simulink model "SIMULACION_LTI_Aumentado"  (R2023b)
settings: Solver=VariableStepAuto  StartTime=0.0  StopTime=2  RelTol=1e-3
values from neighbouring files (symbols this model uses):
  lambda_m = 0.016    [parametros_proyecto2.m]
  Ld = 6.6e-3    (= 0.0066)    [parametros_proyecto2.m]
  Lls = 0.8e-3    (= 0.0008)    [parametros_proyecto2.m]
  Lq = 5.8e-3    (= 0.0058)    [parametros_proyecto2.m]
  r = 120    [parametros_proyecto2.m]
  Rs_ref = 1.02    [parametros_proyecto2.m]
  Rts_amb = 146.7    [parametros_proyecto2.m]
undefined symbols (not defined in the file or in its folder): b_eq, cts, J_eq, P_p, R_s
settings Model: Creator=ignab  LastModifiedBy=ignab

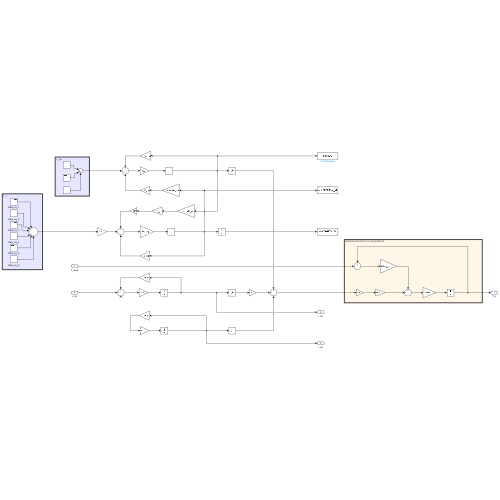
[thumbnail: Simulink's stored preview of the top-level diagram]
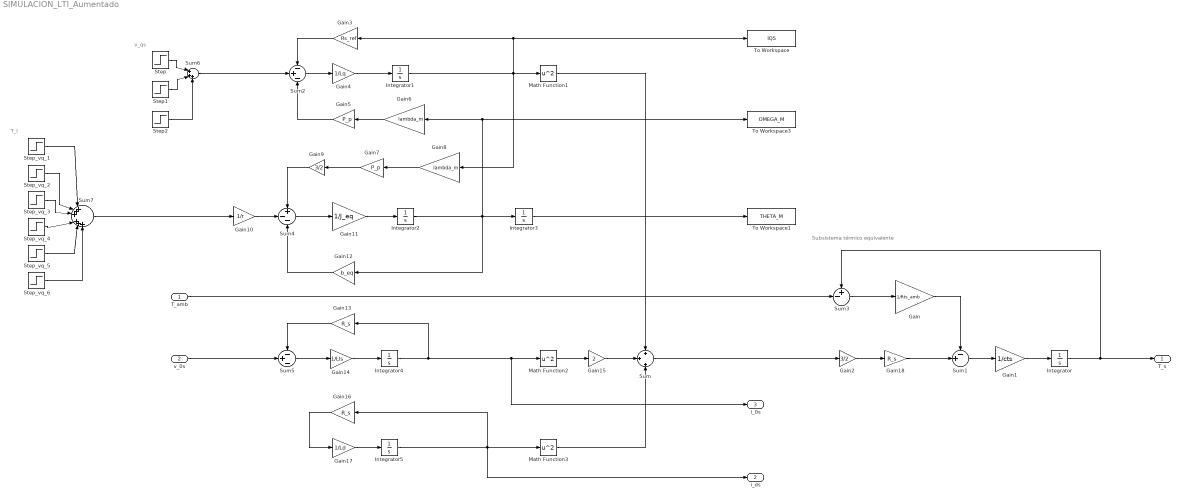
== system SIMULACION_LTI_Aumentado ==
  note: T_l
  note: v_qs
  note: Subsistema térmico equivalente
  T_amb : Inport
  v_0s : Inport  Port=2
  Gain : Gain  Gain=1/Rts_amb
  Gain1 : Gain  Gain=1/cts
  Gain10 : Gain  Gain=1/r
  Gain11 : Gain  Gain=1/J_eq
  Gain12 : Gain  Gain=b_eq
  Gain13 : Gain  Gain=R_s
  Gain14 : Gain  Gain=1/Lls
  Gain15 : Gain  Gain=2
  Gain16 : Gain  Gain=R_s
  Gain17 : Gain  Gain=1/Ld
  Gain18 : Gain  Gain=R_s
  Gain2 : Gain  Gain=3/2
  Gain3 : Gain  Gain=Rs_ref
  Gain4 : Gain  Gain=1/Lq
  Gain5 : Gain  Gain=P_p
  Gain6 : Gain  Gain=lambda_m
  Gain7 : Gain  Gain=P_p
  Gain8 : Gain  Gain=lambda_m
  Gain9 : Gain  Gain=3/2
  Integrator{,1..5} (6 alike) : Integrator
  Math Function1 : Math  Operator=square
  Math Function2 : Math  Operator=square
  Math Function3 : Math  Operator=square
  Step : Step  Time=0.1  After=19.596  SampleTime=0
  Step1 : Step  Time=0.7  After=-39.192  SampleTime=0
  Step2 : Step  Time=1.1  After=19.596  SampleTime=0
  Step_vq_1 : Step  Time=0.3  After=6.28  SampleTime=0
  Step_vq_2 : Step  Time=0.5  After=-12.59  SampleTime=0
  Step_vq_3 : Step  Time=0.9  After=6.28  SampleTime=0
  Step_vq_4 : Step  Time=1.3  After=6.28  SampleTime=0
  Step_vq_5 : Step  Time=1.5  After=-12.59  SampleTime=0
  Step_vq_6 : Step  Time=1.9  After=6.28  SampleTime=0
  Sum : Sum  Inputs=+|+|+
  Sum1 : Sum  Inputs=-+|
  Sum2 : Sum  Inputs=-+-
  Sum3 : Sum  Inputs=+-|
  Sum4 : Sum  Inputs=+--
  Sum5 : Sum  Inputs=-+-
  Sum6 : Sum  Inputs=|+++
  Sum7 : Sum  Inputs=|+++|+++
  To Workspace : ToWorkspace  VariableName=IQS  SaveFormat=Timeseries  SampleTime=-1
      settings: Decimation=2
  To Workspace1 : ToWorkspace  VariableName=THETA_M  SaveFormat=Timeseries  SampleTime=-1
  To Workspace3 : ToWorkspace  VariableName=OMEGA_M  SaveFormat=Timeseries  SampleTime=-1
  T_s : Outport
  i_ds : Outport  Port=2
  i_0s : Outport  Port=3
  wires:
  T_amb/1 -> Sum3/2
  Sum3/1 -> Gain/1
  Gain/1 -> Sum1/1
  Sum1/1 -> Gain1/1
  Gain1/1 -> Integrator/1
  Integrator/1 -> T_s/1, Sum3/1
  Sum6/1 -> Sum2/2
  Gain5/1 -> Sum2/3
  Gain3/1 -> Sum2/1
  Sum2/1 -> Gain4/1
  Gain4/1 -> Integrator1/1
  Gain6/1 -> Gain5/1
  Integrator1/1 -> To Workspace/1, Gain3/1, Math Function1/1, Gain8/1
  Gain8/1 -> Gain7/1
  Gain7/1 -> Gain9/1
  Gain9/1 -> Sum4/1
  Gain12/1 -> Sum4/3
  Sum4/1 -> Gain11/1
  Gain11/1 -> Integrator2/1
  Integrator2/1 -> Integrator3/1, Gain12/1, To Workspace3/1, Gain6/1
  Gain10/1 -> Sum4/2
  Sum7/1 -> Gain10/1
  Integrator4/1 -> i_0s/1, Math Function2/1, Gain13/1
  v_0s/1 -> Sum5/2
  Sum5/1 -> Gain14/1
  Gain14/1 -> Integrator4/1
  Gain13/1 -> Sum5/1
  Gain17/1 -> Integrator5/1
  Gain16/1 -> Gain17/1
  Integrator5/1 -> Gain16/1, Math Function3/1, i_ds/1
  Math Function2/1 -> Gain15/1
  Gain15/1 -> Sum/2
  Math Function1/1 -> Sum/1
  Math Function3/1 -> Sum/3
  Sum/1 -> Gain2/1
  Gain2/1 -> Gain18/1
  Gain18/1 -> Sum1/2
  Integrator3/1 -> To Workspace1/1
  Step2/1 -> Sum6/3
  Step/1 -> Sum6/1
  Step1/1 -> Sum6/2
  Step_vq_1/1 -> Sum7/1
  Step_vq_2/1 -> Sum7/2
  Step_vq_3/1 -> Sum7/3
  Step_vq_4/1 -> Sum7/4
  Step_vq_5/1 -> Sum7/5
  Step_vq_6/1 -> Sum7/6
